simulink model "lab1_sim"  (R2019b)
settings: Solver=ode45  StartTime=0.0  StopTime=Tfin  MaxStep=my_step  RelTol=1e-3
values from neighbouring files (symbols this model uses):
  x0 = [0.01; 0; 0]    [lab_1_ex_2.m]
  xp0 = [0.01; 0.01; 0]    [lab_1_ex_2.m]
settings Model: Creator=user  LastModifiedBy=user

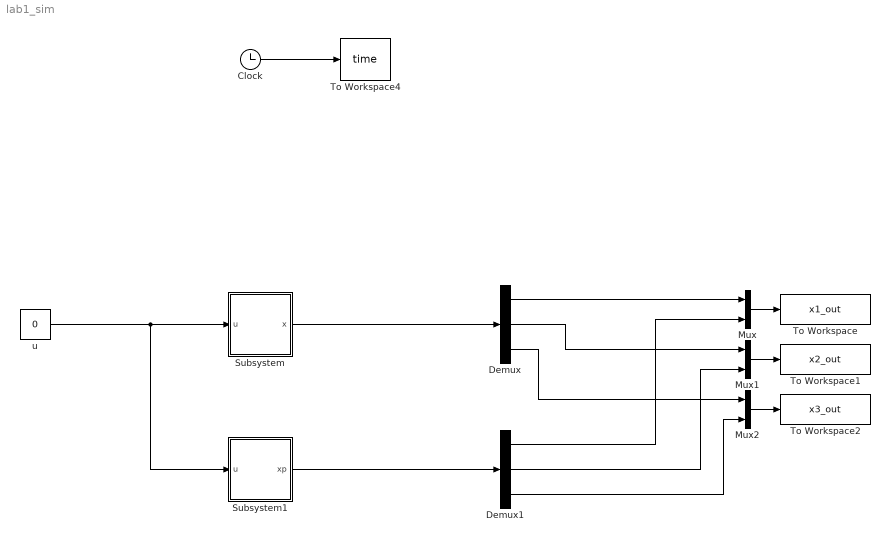
== system lab1_sim ==
  Clock : Clock
  Demux : Demux  Outputs=3
  Demux1 : Demux  Outputs=3
  Mux : Mux  Inputs=2
  Mux1 : Mux  Inputs=2
  Mux2 : Mux  Inputs=2
  Subsystem : Subsystem
  Subsystem1 : Subsystem
  To Workspace : ToWorkspace  VariableName=x1_out  SampleTime=-1
  To Workspace1 : ToWorkspace  VariableName=x2_out  SampleTime=-1
  To Workspace2 : ToWorkspace  VariableName=x3_out  SampleTime=-1
  To Workspace4 : ToWorkspace  VariableName=time  SampleTime=-1
  u : Constant  Value=0
  wires:
  Demux/1 -> Mux/1
  Demux/2 -> Mux1/1
  Demux/3 -> Mux2/1
  Clock/1 -> To Workspace4/1
  u/1 -> Subsystem1/1(u), Subsystem/1(u)
  Subsystem/1(x) -> Demux/1
  Subsystem1/1(xp) -> Demux1/1
  Mux/1 -> To Workspace/1
  Mux1/1 -> To Workspace1/1
  Mux2/1 -> To Workspace2/1
  Demux1/1 -> Mux/2
  Demux1/2 -> Mux1/2
  Demux1/3 -> Mux2/2

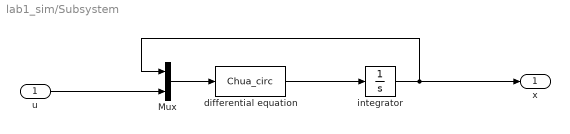
== system lab1_sim/Subsystem ==
  u : Inport
  Mux : Mux  Inputs=2
  differential equation : MATLABFcn  MATLABFcn=Chua_circ
  integrator : Integrator  InitialCondition=x0
  x : Outport
  wires:
  differential equation/1 -> integrator/1
  integrator/1 -> x/1, Mux/1
  u/1 -> Mux/2
  Mux/1 -> differential equation/1

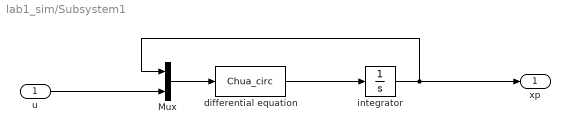
== system lab1_sim/Subsystem1 ==
  u : Inport
  Mux : Mux  Inputs=2
  differential equation : MATLABFcn  MATLABFcn=Chua_circ
  integrator : Integrator  InitialCondition=xp0
  xp : Outport
  wires:
  differential equation/1 -> integrator/1
  integrator/1 -> xp/1, Mux/1
  u/1 -> Mux/2
  Mux/1 -> differential equation/1
